simulink model "Modele_Non_Lineaire"  (R2024a)
settings: Solver=VariableStepAuto  StartTime=0.0  StopTime=10  RelTol=1e-3
values from neighbouring files (symbols this model uses):
  g = 9.81    [Initialisation.m]
  L = 0.4254    [Initialisation.m]
  r_arm = 0.0254    [Initialisation.m]
undefined symbols (not defined in the file or in its folder): den, num
settings Model: Creator=Mathys  LastModifiedBy=francoisdesautels
settings RTWCC: GPUComputeCapability=3.5

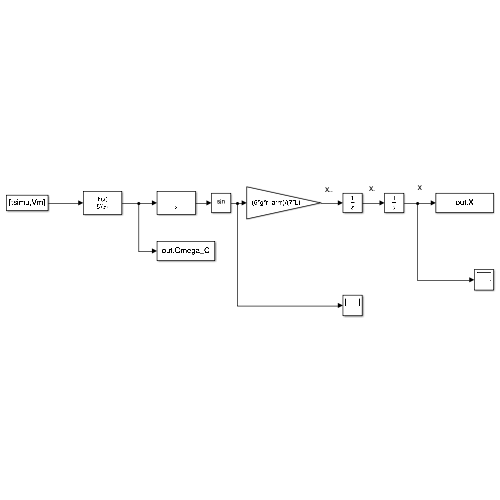
[thumbnail: Simulink's stored preview of the top-level diagram]
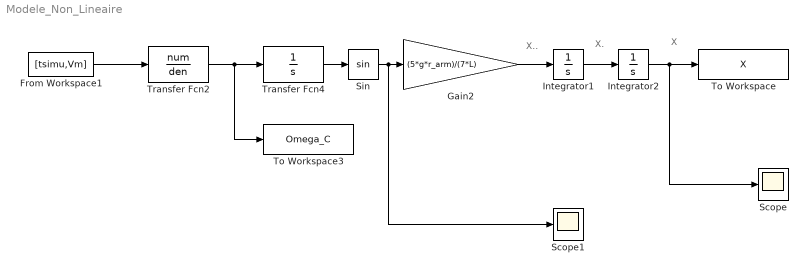
== system Modele_Non_Lineaire ==
  note: X
  note: X.
  note: X..
  From Workspace1 : FromWorkspace  VariableName=[tsimu,Vm]  SampleTime=-1
  Gain2 : Gain  Gain=(5*g*r_arm)/(7*L)
  Integrator1 : Integrator
  Integrator2 : Integrator
  Scope : Scope
  Scope1 : Scope
  Sin : Trigonometry
  To Workspace : ToWorkspace  VariableName=X  SaveFormat=Timeseries  SampleTime=-1
  To Workspace3 : ToWorkspace  VariableName=Omega_C  SampleTime=-1
  Transfer Fcn2 : TransferFcn  Numerator=num  Denominator=den
  Transfer Fcn4 : TransferFcn  Denominator=[1 0]
  wires:
  Sin/1 -> Scope1/1, Gain2/1
  Gain2/1 -> Integrator1/1
  Integrator1/1 -> Integrator2/1
  Integrator2/1 -> Scope/1, To Workspace/1
  Transfer Fcn2/1 -> To Workspace3/1, Transfer Fcn4/1
  From Workspace1/1 -> Transfer Fcn2/1
  Transfer Fcn4/1 -> Sin/1
